simulink model "MotorDC"  (R2014a)
settings: Solver=ode45  StartTime=0.0  StopTime=10.0  RelTol=1e-3
values from neighbouring files (symbols this model uses):
  Ki = 0.2103    [modeladomotorfinal.m]
undefined symbols (not defined in the file or in its folder): B, In, Kv, L, R, Vi
settings Model: Creator=Eladio  LastModifiedBy=Eladio

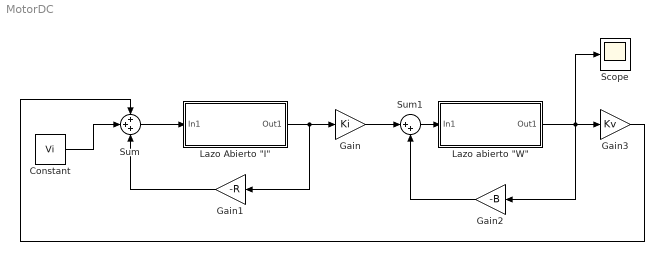
== system MotorDC ==
  Constant : Constant  Value=Vi
  Gain : Gain  Gain=Ki
  Gain1 : Gain  Gain=-R
  Gain2 : Gain  Gain=-B
  Gain3 : Gain  Gain=Kv
  "Lazo Abierto \"I\"" : Subsystem
  "Lazo abierto \"W\"" : Subsystem
  Scope : Scope
  Sum : Sum  Inputs=+++
  Sum1 : Sum  Inputs=|++
  wires:
  Sum/1 -> "Lazo Abierto \"I\""/1(In1)
  "Lazo Abierto \"I\""/1(Out1) -> Gain1/1, Gain/1
  Gain1/1 -> Sum/3
  Constant/1 -> Sum/2
  Sum1/1 -> "Lazo abierto \"W\""/1(In1)
  "Lazo abierto \"W\""/1(Out1) -> Scope/1, Gain2/1, Gain3/1
  Gain3/1 -> Sum/1
  Gain2/1 -> Sum1/2
  Gain/1 -> Sum1/1

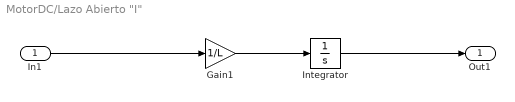
== system MotorDC/Lazo Abierto "I" ==
  In1 : Inport
  Gain1 : Gain  Gain=1/L
  Integrator : Integrator
  Out1 : Outport
  wires:
  Gain1/1 -> Integrator/1
  Integrator/1 -> Out1/1
  In1/1 -> Gain1/1

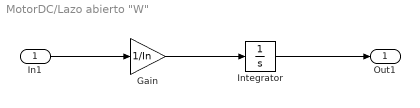
== system MotorDC/Lazo abierto "W" ==
  In1 : Inport
  Gain : Gain  Gain=1/In
  Integrator : Integrator
  Out1 : Outport
  wires:
  Gain/1 -> Integrator/1
  Integrator/1 -> Out1/1
  In1/1 -> Gain/1
